simulink model "PRACTICAL_ASSIGNMENT_02"  (R2025a)
settings: Solver=VariableStepAuto  StartTime=0.0  StopTime=10.0  RelTol=1e-3
settings Model: Creator=nikul  LastModifiedBy=nikul

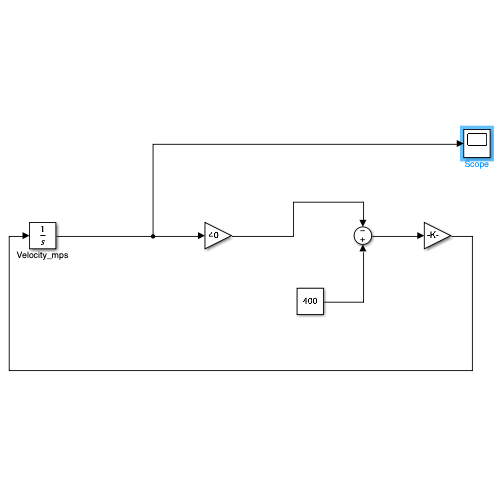
[thumbnail: Simulink's stored preview of the top-level diagram]
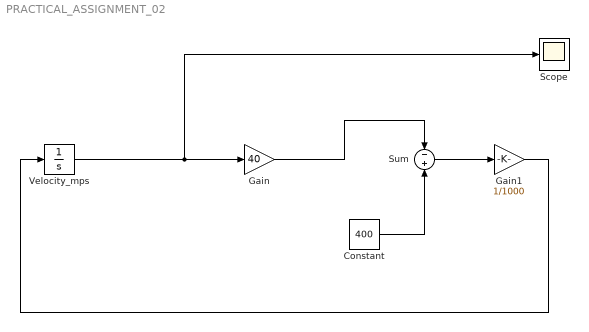
== system PRACTICAL_ASSIGNMENT_02 ==
  Constant : Constant  Value=400
  Gain : Gain  Gain=40
  Gain1 : Gain  Gain=1/1000
  Scope : Scope
      settings: ActiveDisplayYMinimum=0.73273760058397741  ActiveDisplayYMaximum=3.6097479691713263
  Sum : Sum  Inputs=-+
  Velocity_mps : Integrator
  wires:
  Velocity_mps/1 -> Gain/1, Scope/1
  Sum/1 -> Gain1/1
  Gain1/1 -> Velocity_mps/1
  Gain/1 -> Sum/1
  Constant/1 -> Sum/2
